simulink subsystem "SubSystemMotorConveyor"  (R2020b)
settings: Solver=VariableStepAuto  StartTime=0.0  StopTime=10.0  RelTol=1e-3
settings Model: Creator=kaebi  LastModifiedBy=kaebi

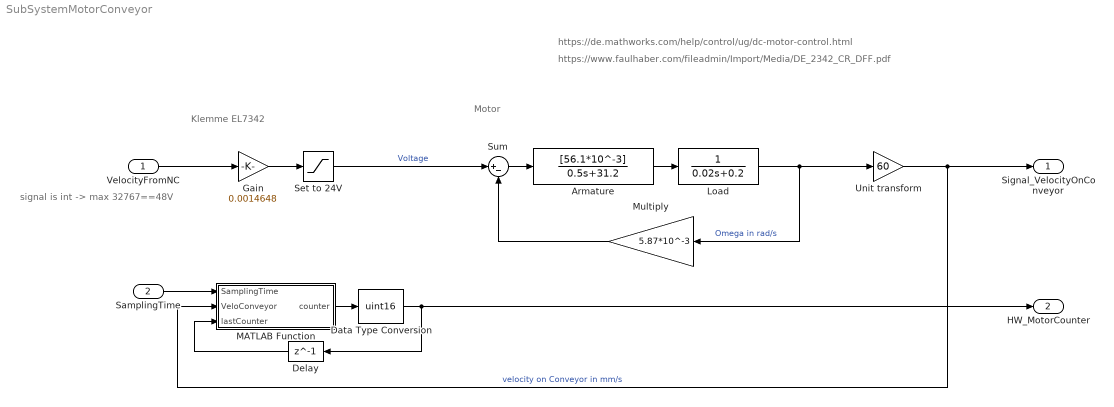
== system SubSystemMotorConveyor ==
  note: Klemme EL7342
  note: Motor
  note: https://www.faulhaber.com/fileadmin/Import/Media/DE_2342_CR_DFF.pdf
  note: https://de.mathworks.com/help/control/ug/dc-motor-control.html
  note: signal is int -> max 32767==48V
  VelocityFromNC : Inport
  SamplingTime : Inport  Port=2
  Armature : TransferFcn  Numerator=[56.1*10^-3]  Denominator=[0.5 31.2]
  Data Type Conversion : DataTypeConversion  OutDataTypeStr=uint16  SaturateOnIntegerOverflow=on
  Delay : Delay  DelayLength=1
  Gain : Gain  Gain=0.0014648
  Load : TransferFcn  Denominator=[0.02 0.2]
  MATLAB Function : MATLAB Function  TreatAsAtomicUnit=on
  Multiply : Gain  Gain=5.87*10^-3
  Set to 24V : Saturate  UpperLimit=24  LowerLimit=-24
  Sum : Sum  Inputs=|+-
  Unit transform : Gain  Gain=60
  Signal_VelocityOnConveyor : Outport
  HW_MotorCounter : Outport  Port=2
  wires:
  Delay/1 -> MATLAB Function/3(lastCounter)
  Data Type Conversion/1 -> Delay/1, HW_MotorCounter/1
  Armature/1 -> Load/1
  Load/1 -> Multiply/1, Unit transform/1  "Omega in rad/s"
  Sum/1 -> Armature/1
  Multiply/1 -> Sum/2
  Unit transform/1 -> Signal_VelocityOnConveyor/1, MATLAB Function/2(VeloConveyor)  "velocity on Conveyor in mm/s"
  VelocityFromNC/1 -> Gain/1
  Gain/1 -> Set to 24V/1
  SamplingTime/1 -> MATLAB Function/1(SamplingTime)
  MATLAB Function/1(counter) -> Data Type Conversion/1
  Set to 24V/1 -> Sum/1  "Voltage"

== matlab function SubSystemMotorConveyor/MATLAB Function ==
  data: SamplingTime input; VeloConveyor input; counter output; lastCounter input
function counter = fcn(SamplingTime, VeloConveyor, lastCounter)
%%
%    VeloConveyor in mm/s
%    SamplingTime in s
%    lastCounter 1count = 0.0001mm

%%

diff = VeloConveyor*SamplingTime*10000;
if (lastCounter+diff >= 65535)
    counter = lastCounter+diff -65535;
else
    counter = lastCounter + VeloConveyor*SamplingTime*10000;
end

end
